simulink model "KillerWhaleModelPneumaticControl"  (R2020b)
settings: Solver=ode15s  StartTime=0.0  StopTime=10  MaxStep=0.01  RelTol=1e-3
model workspace: external: MATLAB File KillerWhaleParams.m (data not in the file)
undefined symbols (not defined in the file or in its folder): frontParams, rearParams, standParams, X, Y, Z
libraries: sm_lib x4301, nesl_utility x6
(part 2 of 66)

== system KillerWhaleModelPneumaticControl/WhaleStand ==
  J5 : Inport
  Cylindrical1 : sm_lib/Joints/Cylindrical Joint  JointMode=Normal  SenseConstraintForce=off  SenseConstraintForceX=off  SenseConstraintForceY=off  SenseConstraintForceZ=off  SenseConstraintTorque=off  SenseConstraintTorqueX=off  SenseConstraintTorqueY=off  SenseConstraintTorqueZ=off  SenseTotalForce=off  SenseTotalForceX=off  SenseTotalForceY=off  SenseTotalForceZ=off  SenseTotalTorque=off  SenseTotalTorqueX=off  SenseTotalTorqueY=off  SenseTotalTorqueZ=off  CompositeWrenchDir=FollowerOnBase  CompositeWrenchFrame=BaseFrame  PzEquilibriumPosition=0  PzEquilibriumPositionUnits=m  PzSpringStiffness=0  PzSpringStiffnessUnits=N/m  PzDampingCoefficient=0  PzDampingCoefficientUnits=N/(m/s)  PzTorqueActuationMode=NoTorque  PzMotionActuationMode=ComputedMotion  PzSensePosition=off  PzSenseVelocity=off  PzSenseAcceleration=off  PzSenseTorqueForce=off  PzSenseLowerLimitTorqueForce=off  PzSenseUpperLimitTorqueForce=off  PzLowerLimitSpecify=off  PzLowerLimitBound=-1  PzLowerLimitBoundUnits=m  PzLowerLimitStiffness=1e6  PzLowerLimitStiffnessUnits=N/m  PzLowerLimitDamping=1e3  PzLowerLimitDampingUnits=N/(m/s)  PzLowerLimitTransitionRegionWidth=1e-4  PzLowerLimitTransitionRegionWidthUnits=m  PzUpperLimitSpecify=off  PzUpperLimitBound=1  PzUpperLimitBoundUnits=m  PzUpperLimitStiffness=1e6  PzUpperLimitStiffnessUnits=N/m  PzUpperLimitDamping=1e3  PzUpperLimitDampingUnits=N/(m/s)  PzUpperLimitTransitionRegionWidth=1e-4  PzUpperLimitTransitionRegionWidthUnits=m  PzPositionTargetSpecify=off  PzPositionTargetPriority=High  PzPositionTargetValue=0  PzPositionTargetValueUnits=m  PzVelocityTargetSpecify=off  PzVelocityTargetPriority=High  PzVelocityTargetValue=0  PzVelocityTargetValueUnits=m/s  RzEquilibriumPosition=0  RzEquilibriumPositionUnits=deg  RzSpringStiffness=0  RzSpringStiffnessUnits=N*m/deg  RzDampingCoefficient=0  RzDampingCoefficientUnits=N*m/(deg/s)  RzTorqueActuationMode=NoTorque  RzMotionActuationMode=ComputedMotion  RzSensePosition=off  RzSenseVelocity=off  RzSenseAcceleration=off  RzSenseTorqueForce=off  RzSenseLowerLimitTorqueForce=off  RzSenseUpperLimitTorqueForce=off  RzLowerLimitSpecify=off  RzLowerLimitBound=-90  RzLowerLimitBoundUnits=deg  RzLowerLimitStiffness=1e4  RzLowerLimitStiffnessUnits=N*m/deg  RzLowerLimitDamping=10  RzLowerLimitDampingUnits=N*m/(deg/s)  RzLowerLimitTransitionRegionWidth=0.1  RzLowerLimitTransitionRegionWidthUnits=deg  RzUpperLimitSpecify=off  RzUpperLimitBound=90  RzUpperLimitBoundUnits=deg  RzUpperLimitStiffness=1e4  RzUpperLimitStiffnessUnits=N*m/deg  RzUpperLimitDamping=10  RzUpperLimitDampingUnits=N*m/(deg/s)  RzUpperLimitTransitionRegionWidth=0.1  RzUpperLimitTransitionRegionWidthUnits=deg  RzPositionTargetSpecify=off  RzPositionTargetPriority=High  RzPositionTargetValue=0  RzPositionTargetValueUnits=deg  RzVelocityTargetSpecify=off  RzVelocityTargetPriority=High  RzVelocityTargetValue=0  RzVelocityTargetValueUnits=deg/s
  Cylindrical2 : sm_lib/Joints/Cylindrical Joint  JointMode=Normal  SenseConstraintForce=off  SenseConstraintForceX=off  SenseConstraintForceY=off  SenseConstraintForceZ=off  SenseConstraintTorque=off  SenseConstraintTorqueX=off  SenseConstraintTorqueY=off  SenseConstraintTorqueZ=off  SenseTotalForce=off  SenseTotalForceX=off  SenseTotalForceY=off  SenseTotalForceZ=off  SenseTotalTorque=off  SenseTotalTorqueX=off  SenseTotalTorqueY=off  SenseTotalTorqueZ=off  CompositeWrenchDir=FollowerOnBase  CompositeWrenchFrame=BaseFrame  PzEquilibriumPosition=0  PzEquilibriumPositionUnits=m  PzSpringStiffness=0  PzSpringStiffnessUnits=N/m  PzDampingCoefficient=0  PzDampingCoefficientUnits=N/(m/s)  PzTorqueActuationMode=NoTorque  PzMotionActuationMode=ComputedMotion  PzSensePosition=off  PzSenseVelocity=off  PzSenseAcceleration=off  PzSenseTorqueForce=off  PzSenseLowerLimitTorqueForce=off  PzSenseUpperLimitTorqueForce=off  PzLowerLimitSpecify=off  PzLowerLimitBound=-1  PzLowerLimitBoundUnits=m  PzLowerLimitStiffness=1e6  PzLowerLimitStiffnessUnits=N/m  PzLowerLimitDamping=1e3  PzLowerLimitDampingUnits=N/(m/s)  PzLowerLimitTransitionRegionWidth=1e-4  PzLowerLimitTransitionRegionWidthUnits=m  PzUpperLimitSpecify=off  PzUpperLimitBound=1  PzUpperLimitBoundUnits=m  PzUpperLimitStiffness=1e6  PzUpperLimitStiffnessUnits=N/m  PzUpperLimitDamping=1e3  PzUpperLimitDampingUnits=N/(m/s)  PzUpperLimitTransitionRegionWidth=1e-4  PzUpperLimitTransitionRegionWidthUnits=m  PzPositionTargetSpecify=off  PzPositionTargetPriority=High  PzPositionTargetValue=0  PzPositionTargetValueUnits=m  PzVelocityTargetSpecify=off  PzVelocityTargetPriority=High  PzVelocityTargetValue=0  PzVelocityTargetValueUnits=m/s  RzEquilibriumPosition=0  RzEquilibriumPositionUnits=deg  RzSpringStiffness=0  RzSpringStiffnessUnits=N*m/deg  RzDampingCoefficient=0  RzDampingCoefficientUnits=N*m/(deg/s)  RzTorqueActuationMode=NoTorque  RzMotionActuationMode=ComputedMotion  RzSensePosition=off  RzSenseVelocity=off  RzSenseAcceleration=off  RzSenseTorqueForce=off  RzSenseLowerLimitTorqueForce=off  RzSenseUpperLimitTorqueForce=off  RzLowerLimitSpecify=off  RzLowerLimitBound=-90  RzLowerLimitBoundUnits=deg  RzLowerLimitStiffness=1e4  RzLowerLimitStiffnessUnits=N*m/deg  RzLowerLimitDamping=10  RzLowerLimitDampingUnits=N*m/(deg/s)  RzLowerLimitTransitionRegionWidth=0.1  RzLowerLimitTransitionRegionWidthUnits=deg  RzUpperLimitSpecify=off  RzUpperLimitBound=90  RzUpperLimitBoundUnits=deg  RzUpperLimitStiffness=1e4  RzUpperLimitStiffnessUnits=N*m/deg  RzUpperLimitDamping=10  RzUpperLimitDampingUnits=N*m/(deg/s)  RzUpperLimitTransitionRegionWidth=0.1  RzUpperLimitTransitionRegionWidthUnits=deg  RzPositionTargetSpecify=off  RzPositionTargetPriority=High  RzPositionTargetValue=0  RzPositionTargetValueUnits=deg  RzVelocityTargetSpecify=off  RzVelocityTargetPriority=High  RzVelocityTargetValue=0  RzVelocityTargetValueUnits=deg/s
  Link_1_1 : Subsystem
  PitchLink2_1 : Subsystem
  PitchLink3_1 : Subsystem
      settings: PortSchema="{\"entries\":[{\"content\":{\"sides\":[{\"content\":{\"connectorIds\":[\"LConn1\"]},\"type\":\"ConnectorPlacement.EquallySpacedRectSide\",\"uuid\":\"a9d62d2a-b569-4d18-acf6-632282cdfd3f\"},{\"content\":{\"connectorIds\":[\"RConn1\"],\"side\":\"RIGHT\"},\"type\":\"ConnectorPlacement.EquallySpacedRectSide\",\"uuid\":\"ddf08f5b-84f7-435f-8135-0f34e66a3f6c\"},{\"content\":{\"connectorIds\":[\"LConn2\"],\"side\":\"TOP\"},\"type\":\"ConnectorPlacement.EquallySpacedRectSide\",\"uuid\":\"528ea33a-f0b8-4f6d-8194-a808427dd81b\"},{\"content\":{\"connectorIds\":[],\"side\":\"HIDDEN\"},\"type\":\"ConnectorPlacement.EquallySpacedRectSide\",\"uuid\":\"99e749ff-748c-40e2-8d76-9e8f4512f99c\"}]},\"type\":\"ConnectorPlacement.EquallySpacedConnector\",\"uuid\":\"82bcbf93-e613-46bd-8073-2373def69e08\"}],\"packageUris\":[\"http://schema.mathworks.com/mf0/Connector/R2020b\"],\"version\":\"1.0\"}"
  PitchLink4_1 : Subsystem
  Revolute1 : sm_lib/Joints/Revolute Joint  JointMode=Normal  SenseConstraintForce=off  SenseConstraintForceX=off  SenseConstraintForceY=off  SenseConstraintForceZ=off  SenseConstraintTorque=off  SenseConstraintTorqueX=off  SenseConstraintTorqueY=off  SenseConstraintTorqueZ=off  SenseTotalForce=off  SenseTotalForceX=off  SenseTotalForceY=off  SenseTotalForceZ=off  SenseTotalTorque=off  SenseTotalTorqueX=off  SenseTotalTorqueY=off  SenseTotalTorqueZ=off  CompositeWrenchDir=FollowerOnBase  CompositeWrenchFrame=BaseFrame  EquilibriumPosition=0  EquilibriumPositionUnits=deg  SpringStiffness=0  SpringStiffnessUnits=N*m/deg  DampingCoefficient=0  DampingCoefficientUnits=N*m/(deg/s)  TorqueActuationMode=NoTorque  MotionActuationMode=ComputedMotion  SensePosition=off  SenseVelocity=off  SenseAcceleration=off  SenseTorqueForce=off  SenseLowerLimitTorqueForce=off  SenseUpperLimitTorqueForce=off  LowerLimitSpecify=off  LowerLimitBound=-90  LowerLimitBoundUnits=deg  LowerLimitStiffness=1e4  LowerLimitStiffnessUnits=N*m/deg  LowerLimitDamping=10  LowerLimitDampingUnits=N*m/(deg/s)  LowerLimitTransitionRegionWidth=0.1  LowerLimitTransitionRegionWidthUnits=deg  UpperLimitSpecify=off  UpperLimitBound=90  UpperLimitBoundUnits=deg  UpperLimitStiffness=1e4  UpperLimitStiffnessUnits=N*m/deg  UpperLimitDamping=10  UpperLimitDampingUnits=N*m/(deg/s)  UpperLimitTransitionRegionWidth=0.1  UpperLimitTransitionRegionWidthUnits=deg  PositionTargetSpecify=on  PositionTargetPriority=Low  PositionTargetValue=standParams.RevoluteJoint(2).Rz.Pos  PositionTargetValueUnits=deg  VelocityTargetSpecify=off  VelocityTargetPriority=High  VelocityTargetValue=0  VelocityTargetValueUnits=deg/s
  Revolute2 : sm_lib/Joints/Revolute Joint  JointMode=Normal  SenseConstraintForce=off  SenseConstraintForceX=off  SenseConstraintForceY=off  SenseConstraintForceZ=off  SenseConstraintTorque=off  SenseConstraintTorqueX=off  SenseConstraintTorqueY=off  SenseConstraintTorqueZ=off  SenseTotalForce=off  SenseTotalForceX=off  SenseTotalForceY=off  SenseTotalForceZ=off  SenseTotalTorque=off  SenseTotalTorqueX=off  SenseTotalTorqueY=off  SenseTotalTorqueZ=off  CompositeWrenchDir=FollowerOnBase  CompositeWrenchFrame=BaseFrame  EquilibriumPosition=0  EquilibriumPositionUnits=deg  SpringStiffness=0  SpringStiffnessUnits=N*m/deg  DampingCoefficient=0  DampingCoefficientUnits=N*m/(deg/s)  TorqueActuationMode=NoTorque  MotionActuationMode=ComputedMotion  SensePosition=off  SenseVelocity=off  SenseAcceleration=off  SenseTorqueForce=off  SenseLowerLimitTorqueForce=off  SenseUpperLimitTorqueForce=off  LowerLimitSpecify=off  LowerLimitBound=-90  LowerLimitBoundUnits=deg  LowerLimitStiffness=1e4  LowerLimitStiffnessUnits=N*m/deg  LowerLimitDamping=10  LowerLimitDampingUnits=N*m/(deg/s)  LowerLimitTransitionRegionWidth=0.1  LowerLimitTransitionRegionWidthUnits=deg  UpperLimitSpecify=off  UpperLimitBound=90  UpperLimitBoundUnits=deg  UpperLimitStiffness=1e4  UpperLimitStiffnessUnits=N*m/deg  UpperLimitDamping=10  UpperLimitDampingUnits=N*m/(deg/s)  UpperLimitTransitionRegionWidth=0.1  UpperLimitTransitionRegionWidthUnits=deg  PositionTargetSpecify=on  PositionTargetPriority=Low  PositionTargetValue=standParams.RevoluteJoint(3).Rz.Pos  PositionTargetValueUnits=deg  VelocityTargetSpecify=off  VelocityTargetPriority=High  VelocityTargetValue=0  VelocityTargetValueUnits=deg/s
  Revolute3 : sm_lib/Joints/Revolute Joint  JointMode=Normal  SenseConstraintForce=off  SenseConstraintForceX=off  SenseConstraintForceY=off  SenseConstraintForceZ=off  SenseConstraintTorque=off  SenseConstraintTorqueX=off  SenseConstraintTorqueY=off  SenseConstraintTorqueZ=off  SenseTotalForce=off  SenseTotalForceX=off  SenseTotalForceY=off  SenseTotalForceZ=off  SenseTotalTorque=off  SenseTotalTorqueX=off  SenseTotalTorqueY=off  SenseTotalTorqueZ=off  CompositeWrenchDir=FollowerOnBase  CompositeWrenchFrame=BaseFrame  EquilibriumPosition=0  EquilibriumPositionUnits=deg  SpringStiffness=0  SpringStiffnessUnits=N*m/deg  DampingCoefficient=0  DampingCoefficientUnits=N*m/(deg/s)  TorqueActuationMode=NoTorque  MotionActuationMode=ComputedMotion  SensePosition=off  SenseVelocity=off  SenseAcceleration=off  SenseTorqueForce=off  SenseLowerLimitTorqueForce=off  SenseUpperLimitTorqueForce=off  LowerLimitSpecify=off  LowerLimitBound=-90  LowerLimitBoundUnits=deg  LowerLimitStiffness=1e4  LowerLimitStiffnessUnits=N*m/deg  LowerLimitDamping=10  LowerLimitDampingUnits=N*m/(deg/s)  LowerLimitTransitionRegionWidth=0.1  LowerLimitTransitionRegionWidthUnits=deg  UpperLimitSpecify=off  UpperLimitBound=90  UpperLimitBoundUnits=deg  UpperLimitStiffness=1e4  UpperLimitStiffnessUnits=N*m/deg  UpperLimitDamping=10  UpperLimitDampingUnits=N*m/(deg/s)  UpperLimitTransitionRegionWidth=0.1  UpperLimitTransitionRegionWidthUnits=deg  PositionTargetSpecify=on  PositionTargetPriority=Low  PositionTargetValue=standParams.RevoluteJoint(5).Rz.Pos  PositionTargetValueUnits=deg  VelocityTargetSpecify=off  VelocityTargetPriority=High  VelocityTargetValue=0  VelocityTargetValueUnits=deg/s
  Revolute4 : sm_lib/Joints/Revolute Joint  JointMode=Normal  SenseConstraintForce=off  SenseConstraintForceX=off  SenseConstraintForceY=off  SenseConstraintForceZ=off  SenseConstraintTorque=off  SenseConstraintTorqueX=off  SenseConstraintTorqueY=off  SenseConstraintTorqueZ=off  SenseTotalForce=off  SenseTotalForceX=off  SenseTotalForceY=off  SenseTotalForceZ=off  SenseTotalTorque=off  SenseTotalTorqueX=off  SenseTotalTorqueY=off  SenseTotalTorqueZ=off  CompositeWrenchDir=FollowerOnBase  CompositeWrenchFrame=BaseFrame  EquilibriumPosition=0  EquilibriumPositionUnits=deg  SpringStiffness=0  SpringStiffnessUnits=N*m/deg  DampingCoefficient=0  DampingCoefficientUnits=N*m/(deg/s)  TorqueActuationMode=NoTorque  MotionActuationMode=ComputedMotion  SensePosition=off  SenseVelocity=off  SenseAcceleration=off  SenseTorqueForce=off  SenseLowerLimitTorqueForce=off  SenseUpperLimitTorqueForce=off  LowerLimitSpecify=off  LowerLimitBound=-90  LowerLimitBoundUnits=deg  LowerLimitStiffness=1e4  LowerLimitStiffnessUnits=N*m/deg  LowerLimitDamping=10  LowerLimitDampingUnits=N*m/(deg/s)  LowerLimitTransitionRegionWidth=0.1  LowerLimitTransitionRegionWidthUnits=deg  UpperLimitSpecify=off  UpperLimitBound=90  UpperLimitBoundUnits=deg  UpperLimitStiffness=1e4  UpperLimitStiffnessUnits=N*m/deg  UpperLimitDamping=10  UpperLimitDampingUnits=N*m/(deg/s)  UpperLimitTransitionRegionWidth=0.1  UpperLimitTransitionRegionWidthUnits=deg  PositionTargetSpecify=on  PositionTargetPriority=Low  PositionTargetValue=standParams.RevoluteJoint(1).Rz.Pos  PositionTargetValueUnits=deg  VelocityTargetSpecify=off  VelocityTargetPriority=High  VelocityTargetValue=0  VelocityTargetValueUnits=deg/s
  Revolute5 : sm_lib/Joints/Revolute Joint  JointMode=Normal  SenseConstraintForce=off  SenseConstraintForceX=off  SenseConstraintForceY=off  SenseConstraintForceZ=off  SenseConstraintTorque=off  SenseConstraintTorqueX=off  SenseConstraintTorqueY=off  SenseConstraintTorqueZ=off  SenseTotalForce=off  SenseTotalForceX=off  SenseTotalForceY=off  SenseTotalForceZ=off  SenseTotalTorque=off  SenseTotalTorqueX=off  SenseTotalTorqueY=off  SenseTotalTorqueZ=off  CompositeWrenchDir=FollowerOnBase  CompositeWrenchFrame=BaseFrame  EquilibriumPosition=0  EquilibriumPositionUnits=deg  SpringStiffness=0  SpringStiffnessUnits=N*m/deg  DampingCoefficient=0  DampingCoefficientUnits=N*m/(deg/s)  TorqueActuationMode=NoTorque  MotionActuationMode=ComputedMotion  SensePosition=off  SenseVelocity=off  SenseAcceleration=off  SenseTorqueForce=off  SenseLowerLimitTorqueForce=off  SenseUpperLimitTorqueForce=off  LowerLimitSpecify=off  LowerLimitBound=-90  LowerLimitBoundUnits=deg  LowerLimitStiffness=1e4  LowerLimitStiffnessUnits=N*m/deg  LowerLimitDamping=10  LowerLimitDampingUnits=N*m/(deg/s)  LowerLimitTransitionRegionWidth=0.1  LowerLimitTransitionRegionWidthUnits=deg  UpperLimitSpecify=off  UpperLimitBound=90  UpperLimitBoundUnits=deg  UpperLimitStiffness=1e4  UpperLimitStiffnessUnits=N*m/deg  UpperLimitDamping=10  UpperLimitDampingUnits=N*m/(deg/s)  UpperLimitTransitionRegionWidth=0.1  UpperLimitTransitionRegionWidthUnits=deg  PositionTargetSpecify=on  PositionTargetPriority=Low  PositionTargetValue=standParams.RevoluteJoint(4).Rz.Pos  PositionTargetValueUnits=deg  VelocityTargetSpecify=off  VelocityTargetPriority=High  VelocityTargetValue=0  VelocityTargetValueUnits=deg/s
  Stand_1 : Subsystem
  Stand_Actuator_1 : Subsystem
      settings: PortSchema="{\"entries\":[{\"content\":{\"sides\":[{\"content\":{\"connectorIds\":[\"LConn1\"]},\"type\":\"ConnectorPlacement.EquallySpacedRectSide\",\"uuid\":\"a2790423-1875-4f6c-bcc8-f8951bbf04a9\"},{\"content\":{\"connectorIds\":[\"RConn1\"],\"side\":\"RIGHT\"},\"type\":\"ConnectorPlacement.EquallySpacedRectSide\",\"uuid\":\"c84b9fae-4c29-439d-9486-1840c3d66b05\"},{\"content\":{\"connectorIds\":[\"In1\"],\"side\":\"TOP\"},\"type\":\"ConnectorPlacement.EquallySpacedRectSide\",\"uuid\":\"97f54a40-5d41-49e0-a709-056e005671f1\"},{\"content\":{\"connectorIds\":[],\"side\":\"HIDDEN\"},\"type\":\"ConnectorPlacement.EquallySpacedRectSide\",\"uuid\":\"427997b4-744f-45dd-b609-16314c135bf0\"}]},\"type\":\"ConnectorPlacement.EquallySpacedConnector\",\"uuid\":\"a7b9e3e0-830a-4064-b5fb-feaf5802e4ca\"}],\"packageUris\":[\"http://schema.mathworks.com/mf0/Connector/R2020b\"],\"version\":\"1.0\"}"
  Transform : sm_lib/Frames and Transforms/Rigid Transform  TranslationMethod=Cartesian  TranslationStandardOffset=0  TranslationLengthUnit=in  TranslationStandardAxis=+Z  TranslationCartesianOffset=standParams.RigidTransform(321).translation  TranslationROffset=0  TranslationROffsetUnits=m  TranslationZOffset=0  TranslationZOffsetUnits=m  TranslationThetaOffset=0  TranslationThetaOffsetUnits=deg  RotationMethod=ArbitraryAxis  RotationAngleUnits=rad  RotationStandardAxis=+Z  RotationAngle=standParams.RigidTransform(321).angle  RotationArbitraryAxis=standParams.RigidTransform(321).axis  FollAlignAxisA=+X  BaseAlignAxisA=+Y  FollAlignAxisB=+Y  BaseAlignAxisB=+Z  RotationSequenceAxes=FollowerAxes  RotationSequence=XYX  RotationSequenceAngles=[0 0 0]  RotationSequenceAnglesUnits=deg  RotationMatrix=[1 0 0; 0 1 0; 0 0 1]
  S1 : PMIOPort  Side=Left
  S2 : PMIOPort  Port=2  Side=Left
  wires:
  J5/1 -> Stand_Actuator_1/1(J5)
  connections:
  Cylindrical2/LConn1 -- Stand_Actuator_1/RConn1
  Revolute5/RConn1 -- Stand_Actuator_1/LConn1
  Cylindrical1/RConn1 -- Link_1_1/LConn2
  PitchLink3_1/LConn1 -- Revolute3/RConn1
  PitchLink3_1/RConn1 -- Revolute1/LConn1
  Revolute5/LConn1 -- Stand_1/RConn1
  PitchLink4_1/LConn1 -- Revolute4/RConn1
  PitchLink2_1/RConn2 -- Revolute2/LConn1
  Cylindrical2/RConn1 -- Link_1_1/LConn1
  Cylindrical1/LConn1 -- Stand_1/RConn2
  Transform/RConn1 -- Stand_1/LConn1
  Revolute4/LConn1 -- Stand_1/RConn3
  PitchLink4_1/LConn2 -- Revolute1/RConn1
  Link_1_1/LConn3 -- Revolute2/RConn1
  PitchLink2_1/RConn1 -- Revolute3/LConn1
  S2/RConn1 -- Transform/LConn1
  S1/RConn1 -- PitchLink3_1/LConn2

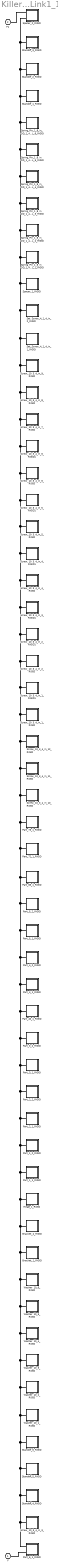
== system KillerWhaleModelPneumaticControl/HeadLinkage/HeadLink1_1 ==
  Bracket_1_RIGID : Subsystem
  Bracket_2_RIGID : Subsystem
  Hinge_1_RIGID : Subsystem
  Part_1_1_RIGID : Subsystem
  Part_1_2_RIGID : Subsystem
  Part_2_1_RIGID : Subsystem
  Part_2_2_RIGID : Subsystem
  Part_3_1_RIGID : Subsystem
  Part_3_2_RIGID : Subsystem
  Part_40_1_RIGID : Subsystem
  Part_4_1_RIGID : Subsystem
  Part_4_2_RIGID : Subsystem
  Part_5_1_RIGID : Subsystem
  Part_5_2_RIGID : Subsystem
  Part_65_1_RIGID : Subsystem
  Part_6_1_RIGID : Subsystem
  Part_72_1_RIGID : Subsystem
  Part_73_1_RIGID : Subsystem
  Screw_10_3_4_in_10_RIGID : Subsystem
  Screw_10_3_4_in_11_RIGID : Subsystem
  Screw_10_3_4_in_12_RIGID : Subsystem
  Screw_10_3_4_in_1_RIGID : Subsystem
  Screw_10_3_4_in_1_RIGID1 : Subsystem
  Screw_10_3_4_in_2_RIGID : Subsystem
  Screw_10_3_4_in_2_RIGID1 : Subsystem
  Screw_10_3_4_in_3_RIGID : Subsystem
  Screw_10_3_4_in_3_RIGID1 : Subsystem
  Screw_10_3_4_in_4_RIGID : Subsystem
  Screw_10_3_4_in_4_RIGID1 : Subsystem
  Screw_10_3_4_in_5_RIGID : Subsystem
  Screw_10_3_4_in_5_RIGID1 : Subsystem
  Screw_10_3_4_in_6_RIGID : Subsystem
  Screw_10_3_4_in_6_RIGID1 : Subsystem
  Screw_10_3_4_in_7_RIGID : Subsystem
  Screw_10_3_4_in_8_RIGID : Subsystem
  Screw_10_3_4_in_9_RIGID : Subsystem
  Set_Screw_4_1_4_in_1_RIGID : Subsystem
  Set_Screw_4_1_4_in_2_RIGID : Subsystem
  Spacer_1_RIGID : Subsystem
  Spacer_2_RIGID : Subsystem
  Spring_Pin_1_8_in_OD_1_4_in_L_1_RIGID : Subsystem
  Spring_Pin_1_8_in_OD_1_4_in_L_2_RIGID : Subsystem
  Spring_Pin_1_8_in_OD_1_4_in_L_3_RIGID : Subsystem
  Spring_Pin_1_8_in_OD_1_4_in_L_4_RIGID : Subsystem
  Spring_Pin_1_8_in_OD_1_4_in_L_5_RIGID : Subsystem
  Spring_Pin_1_8_in_OD_1_4_in_L_6_RIGID : Subsystem
  Standoff_1_RIGID : Subsystem
  Standoff_2_RIGID : Subsystem
  Standoff_3_RIGID : Subsystem
  Standoff_4_RIGID : Subsystem
  Standoff_5_RIGID : Subsystem
  Standoff_6_RIGID : Subsystem
  Washer_10_1_RIGID : Subsystem
  Washer_10_2_RIGID : Subsystem
  Washer_10_3_RIGID : Subsystem
  Washer_10_4_RIGID : Subsystem
  Washer_10_5_RIGID : Subsystem
  Washer_10_6_RIGID : Subsystem
  F : PMIOPort  Side=Left
  F1 : PMIOPort  Port=2  Side=Right
  connections:
  Bracket_1_RIGID/LConn1 -- Part_6_1_RIGID/LConn1 -- Screw_10_3_4_in_3_RIGID/LConn1 -- Standoff_4_RIGID/LConn1 -- Standoff_5_RIGID/LConn1 -- Standoff_6_RIGID/LConn1 -- Washer_10_1_RIGID/LConn1 -- Washer_10_2_RIGID/LConn1 -- Washer_10_3_RIGID/LConn1 -- Washer_10_4_RIGID/LConn1 -- Washer_10_5_RIGID/LConn1 -- Washer_10_6_RIGID/LConn1 -- Spacer_2_RIGID/LConn2 -- Standoff_3_RIGID/LConn1 -- Standoff_2_RIGID/LConn1 -- Standoff_1_RIGID/LConn1 -- Spring_Pin_1_8_in_OD_1_4_in_L_6_RIGID/LConn1 -- Spring_Pin_1_8_in_OD_1_4_in_L_5_RIGID/LConn1 -- Spring_Pin_1_8_in_OD_1_4_in_L_4_RIGID/LConn1 -- Spring_Pin_1_8_in_OD_1_4_in_L_3_RIGID/LConn1 -- Spring_Pin_1_8_in_OD_1_4_in_L_2_RIGID/LConn1 -- Spring_Pin_1_8_in_OD_1_4_in_L_1_RIGID/LConn1 -- Spacer_1_RIGID/LConn1 -- Set_Screw_4_1_4_in_2_RIGID/LConn1 -- Set_Screw_4_1_4_in_1_RIGID/LConn1 -- Screw_10_3_4_in_9_RIGID/LConn1 -- Screw_10_3_4_in_8_RIGID/LConn1 -- Screw_10_3_4_in_7_RIGID/LConn1 -- Screw_10_3_4_in_6_RIGID1/LConn1 -- Screw_10_3_4_in_6_RIGID/LConn1 -- Screw_10_3_4_in_5_RIGID1/LConn1 -- Screw_10_3_4_in_5_RIGID/LConn1 -- Screw_10_3_4_in_4_RIGID1/LConn1 -- Screw_10_3_4_in_4_RIGID/LConn1 -- Screw_10_3_4_in_3_RIGID1/LConn1 -- Screw_10_3_4_in_2_RIGID1/LConn1 -- Screw_10_3_4_in_2_RIGID/LConn1 -- Screw_10_3_4_in_1_RIGID1/LConn1 -- Screw_10_3_4_in_1_RIGID/LConn1 -- Screw_10_3_4_in_12_RIGID/LConn1 -- Screw_10_3_4_in_11_RIGID/LConn1 -- Screw_10_3_4_in_10_RIGID/LConn1 -- Part_73_1_RIGID/LConn1 -- Part_72_1_RIGID/LConn1 -- Part_65_1_RIGID/LConn1 -- Part_5_2_RIGID/LConn1 -- Part_5_1_RIGID/LConn1 -- Part_4_2_RIGID/LConn1 -- Part_4_1_RIGID/LConn1 -- Part_40_1_RIGID/LConn1 -- Part_3_2_RIGID/LConn1 -- Part_3_1_RIGID/LConn1 -- Part_2_2_RIGID/LConn1 -- Part_2_1_RIGID/LConn1 -- Part_1_2_RIGID/LConn1 -- Part_1_1_RIGID/LConn1 -- Hinge_1_RIGID/LConn1 -- Bracket_2_RIGID/LConn1
  Part_6_1_RIGID/LConn2 -- F/RConn1
  Spacer_2_RIGID/LConn1 -- F1/RConn1

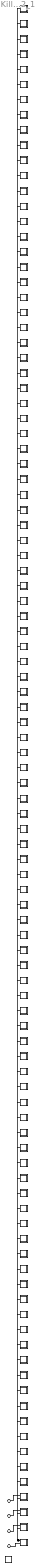
== system KillerWhaleModelPneumaticControl/HeadLinkage/HeadLink2_1 ==
  Frame_Part_1_RIGID : Subsystem
  Frame_Part_2_RIGID : Subsystem
  Part_1_1_RIGID : Subsystem
  Part_1_2_RIGID : Subsystem
  Part_1_3_RIGID : Subsystem
  Part_1_4_RIGID : Subsystem
  Part_24_1_RIGID : Subsystem
  Part_24r_1_RIGID : Subsystem
  Part_2_1_RIGID : Subsystem
  Part_2_2_RIGID : Subsystem
  Part_2_3_RIGID : Subsystem
  Part_2_4_RIGID : Subsystem
  Part_3_1_RIGID : Subsystem
  Part_3_2_RIGID : Subsystem
  Part_3_3_RIGID : Subsystem
  Part_3_4_RIGID : Subsystem
  Part_4_1_RIGID : Subsystem
  Part_4_2_RIGID : Subsystem
  Part_4_3_RIGID : Subsystem
  Part_4_4_RIGID : Subsystem
  Part_5_1_RIGID : Subsystem
  Part_5_2_RIGID : Subsystem
  Part_5_3_RIGID : Subsystem
  Part_5_4_RIGID : Subsystem
  Part_6_1_RIGID : Subsystem
  Part_6_2_RIGID : Subsystem
  Part_809_1_RIGID : Subsystem
  Part_809_2_RIGID : Subsystem
  Part_809_3_RIGID : Subsystem
  Part_809_4_RIGID : Subsystem
  Part_809_5_RIGID : Subsystem
  Part_811_1_RIGID : Subsystem
  Part_812_1_RIGID : Subsystem
  Part_813_1_RIGID : Subsystem
  Part_814_1_RIGID : Subsystem
  Part_815_1_RIGID : Subsystem
  Part_816_1_RIGID : Subsystem
  Part_817_1_RIGID : Subsystem
  Part_818_1_RIGID : Subsystem
  Part_819_1_RIGID : Subsystem
  Part_820_1_RIGID : Subsystem
  Part_821_1_RIGID : Subsystem
  Part_822_1_RIGID : Subsystem
  Part_823_1_RIGID : Subsystem
  Part_824_1_RIGID : Subsystem
  Part_824_2_RIGID : Subsystem
  Part_825_1_RIGID : Subsystem
  Part_825_2_RIGID : Subsystem
  Part_826_1_RIGID : Subsystem
  Part_826_2_RIGID : Subsystem
  Part_827_1_RIGID : Subsystem
  Part_827_2_RIGID : Subsystem
  Part_828_1_RIGID : Subsystem
  Part_828_2_RIGID : Subsystem
  Part_867_1_RIGID : Subsystem
  Part_870_1_RIGID : Subsystem
  Part_875_1_RIGID : Subsystem
  Part_936_1_RIGID : Subsystem
  Part_937_1_RIGID : Subsystem
  Part_938_1_RIGID : Subsystem
  Part_939_1_RIGID : Subsystem
  ReferenceFrame : sm_lib/Frames and Transforms/Reference Frame
  Screw_10_3_4_in_1_RIGID : Subsystem
  Screw_10_3_4_in_2_RIGID : Subsystem
  Screw_10_3_4_in_3_RIGID : Subsystem
  Screw_10_3_4_in_4_RIGID : Subsystem
  Screw_10_3_4_in_5_RIGID : Subsystem
  Screw_10_3_4_in_6_RIGID : Subsystem
  Screw_8_1_2_in_1_RIGID : Subsystem
  Screw_8_1_2_in_2_RIGID : Subsystem
  Spring_Pin_1_8_in_OD_1_4_in_L_1_RIGID : Subsystem
  Spring_Pin_1_8_in_OD_1_4_in_L_2_RIGID : Subsystem
  Spring_Pin_1_8_in_OD_1_4_in_L_3_RIGID : Subsystem
  Spring_Pin_1_8_in_OD_1_4_in_L_4_RIGID : Subsystem
  Spring_Pin_1_8_in_OD_1_4_in_L_5_RIGID : Subsystem
  Spring_Pin_1_8_in_OD_1_4_in_L_6_RIGID : Subsystem
  Standoff_1_RIGID : Subsystem
  Washer_10_10_RIGID : Subsystem
  Washer_10_1_RIGID : Subsystem
  Washer_10_2_RIGID : Subsystem
  Washer_10_3_RIGID : Subsystem
  Washer_10_4_RIGID : Subsystem
  Washer_10_5_RIGID : Subsystem
  Washer_10_6_RIGID : Subsystem
  Washer_10_7_RIGID : Subsystem
  Washer_10_8_RIGID : Subsystem
  Washer_10_9_RIGID : Subsystem
  Washer_8_1_RIGID : Subsystem
  Washer_8_2_RIGID : Subsystem
  bulkheads7_1_RIGID : Subsystem
  bulkheads7_2_RIGID : Subsystem
  bulkheads7_3_RIGID : Subsystem
  bulkheads7_4_RIGID : Subsystem
  bulkheads7_5_RIGID : Subsystem
  bulkheads8_1_RIGID : Subsystem
  bulkheads8_2_RIGID : Subsystem
  bulkheads8_3_RIGID : Subsystem
  bulkheads8_4_RIGID : Subsystem
  bulkheads8_5_RIGID : Subsystem
  nut_1_RIGID : Subsystem
  nut_2_RIGID : Subsystem
  nut_3_RIGID : Subsystem
  nut_4_RIGID : Subsystem
  F2 : PMIOPort  Side=Left
  F1 : PMIOPort  Port=2  Side=Left
  F4 : PMIOPort  Port=3  Side=Right
  F : PMIOPort  Port=4  Side=Right
  connections:
  Frame_Part_1_RIGID/LConn1 -- Frame_Part_2_RIGID/LConn2 -- Part_1_1_RIGID/LConn1 -- Part_1_2_RIGID/LConn1 -- Part_1_3_RIGID/LConn2 -- Part_1_4_RIGID/LConn2 -- Part_24_1_RIGID/LConn1 -- Part_24r_1_RIGID/LConn1 -- Part_2_1_RIGID/LConn1 -- Part_2_2_RIGID/LConn1 -- Part_2_3_RIGID/LConn1 -- Part_2_4_RIGID/LConn1 -- Part_3_1_RIGID/LConn1 -- Part_3_2_RIGID/LConn1 -- Part_3_3_RIGID/LConn1 -- Part_3_4_RIGID/LConn1 -- Part_4_1_RIGID/LConn1 -- Part_4_2_RIGID/LConn1 -- Part_4_3_RIGID/LConn1 -- Part_4_4_RIGID/LConn1 -- Part_5_1_RIGID/LConn1 -- Part_5_2_RIGID/LConn1 -- Part_5_3_RIGID/LConn1 -- Part_5_4_RIGID/LConn1 -- Part_6_1_RIGID/LConn1 -- Part_6_2_RIGID/LConn1 -- Part_809_1_RIGID/LConn1 -- Part_809_2_RIGID/LConn1 -- Part_809_3_RIGID/LConn1 -- Part_809_4_RIGID/LConn1 -- Part_809_5_RIGID/LConn1 -- Part_811_1_RIGID/LConn1 -- Part_812_1_RIGID/LConn1 -- Part_813_1_RIGID/LConn1 -- Part_814_1_RIGID/LConn1 -- Part_815_1_RIGID/LConn1 -- Part_816_1_RIGID/LConn1 -- Part_817_1_RIGID/LConn1 -- Part_818_1_RIGID/LConn1 -- Part_819_1_RIGID/LConn1 -- Part_820_1_RIGID/LConn1 -- Part_821_1_RIGID/LConn1 -- Part_822_1_RIGID/LConn1 -- Part_823_1_RIGID/LConn1 -- Part_824_1_RIGID/LConn1 -- Part_824_2_RIGID/LConn1 -- Part_825_1_RIGID/LConn1 -- Part_825_2_RIGID/LConn1 -- Part_826_1_RIGID/LConn1 -- Part_826_2_RIGID/LConn1 -- Part_827_1_RIGID/LConn1 -- Part_827_2_RIGID/LConn1 -- Part_828_1_RIGID/LConn1 -- Part_828_2_RIGID/LConn1 -- Part_867_1_RIGID/LConn1 -- Part_870_1_RIGID/LConn1 -- Part_875_1_RIGID/LConn1 -- Part_936_1_RIGID/LConn1 -- Part_937_1_RIGID/LConn1 -- Part_938_1_RIGID/LConn1 -- Part_939_1_RIGID/LConn1 -- Screw_10_3_4_in_1_RIGID/LConn1 -- Screw_10_3_4_in_2_RIGID/LConn1 -- Screw_10_3_4_in_3_RIGID/LConn1 -- Screw_10_3_4_in_4_RIGID/LConn1 -- Screw_10_3_4_in_5_RIGID/LConn1 -- Screw_10_3_4_in_6_RIGID/LConn1 -- Screw_8_1_2_in_1_RIGID/LConn1 -- Screw_8_1_2_in_2_RIGID/LConn1 -- Spring_Pin_1_8_in_OD_1_4_in_L_1_RIGID/LConn1 -- Spring_Pin_1_8_in_OD_1_4_in_L_2_RIGID/LConn1 -- Spring_Pin_1_8_in_OD_1_4_in_L_3_RIGID/LConn1 -- Spring_Pin_1_8_in_OD_1_4_in_L_4_RIGID/LConn1 -- Spring_Pin_1_8_in_OD_1_4_in_L_5_RIGID/LConn1 -- Spring_Pin_1_8_in_OD_1_4_in_L_6_RIGID/LConn1 -- Standoff_1_RIGID/LConn1 -- Washer_10_10_RIGID/LConn1 -- Washer_10_1_RIGID/LConn1 -- Washer_10_2_RIGID/LConn1 -- Washer_10_3_RIGID/LConn1 -- Washer_10_4_RIGID/LConn1 -- Washer_10_5_RIGID/LConn1 -- Washer_10_6_RIGID/LConn1 -- Washer_10_7_RIGID/LConn1 -- Washer_10_8_RIGID/LConn1 -- Washer_10_9_RIGID/LConn1 -- Washer_8_1_RIGID/LConn1 -- Washer_8_2_RIGID/LConn1 -- bulkheads7_1_RIGID/LConn1 -- bulkheads7_2_RIGID/LConn1 -- bulkheads7_3_RIGID/LConn1 -- bulkheads7_4_RIGID/LConn1 -- bulkheads7_5_RIGID/LConn1 -- bulkheads8_1_RIGID/LConn1 -- bulkheads8_2_RIGID/LConn1 -- bulkheads8_3_RIGID/LConn1 -- bulkheads8_4_RIGID/LConn1 -- bulkheads8_5_RIGID/LConn1 -- nut_1_RIGID/LConn1 -- nut_2_RIGID/LConn1 -- nut_3_RIGID/LConn1 -- nut_4_RIGID/LConn1
  Part_1_4_RIGID/LConn1 -- F/RConn1
  Frame_Part_1_RIGID/LConn2 -- F1/RConn1
  Frame_Part_2_RIGID/LConn1 -- F2/RConn1
  Part_1_3_RIGID/LConn1 -- F4/RConn1

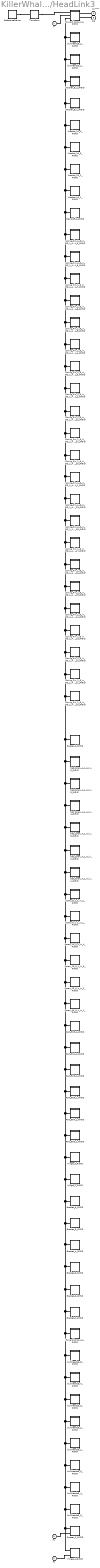
== system KillerWhaleModelPneumaticControl/HeadLinkage/HeadLink3_1 ==
  Bracket_1_RIGID : Subsystem
  Bracket_2_RIGID : Subsystem
  Bracket_3_RIGID : Subsystem
  Bracket_4_RIGID : Subsystem
  Bracket_5_RIGID : Subsystem
  Bracket_6_RIGID : Subsystem
  Hinge_1_RIGID : Subsystem
  Hinge_2_RIGID : Subsystem
  Hinge_3_RIGID : Subsystem
  Part_853_1_RIGID : Subsystem
  Part_854_1_RIGID : Subsystem
  Part_855_1_RIGID : Subsystem
  Part_923_1_RIGID : Subsystem
  Part_924_1_RIGID : Subsystem
  Part_925_1_RIGID : Subsystem
  ReferenceFrame : sm_lib/Frames and Transforms/Reference Frame
  Screw_10_3_4_in_1_RIGID : Subsystem
  Screw_10_3_4_in_2_RIGID : Subsystem
  Screw_10_3_4_in_3_RIGID : Subsystem
  Screw_10_3_4_in_4_RIGID : Subsystem
  Screw_8_1_2_in_1_RIGID : Subsystem
  Screw_8_1_2_in_2_RIGID : Subsystem
  Set_Screw_4_1_4_in_1_RIGID : Subsystem
  Set_Screw_4_1_4_in_2_RIGID : Subsystem
  Set_Screw_4_1_4_in_3_RIGID : Subsystem
  Set_Screw_4_1_4_in_4_RIGID : Subsystem
  Set_Screw_4_1_4_in_5_RIGID : Subsystem
  Set_Screw_4_1_4_in_6_RIGID : Subsystem
  Spacer_1_RIGID : Subsystem
  Spacer_2_RIGID : Subsystem
  Spring_Pin_1_8_in_OD_1_4_in_L_10_RIGID : Subsystem
  Spring_Pin_1_8_in_OD_1_4_in_L_11_RIGID : Subsystem
  Spring_Pin_1_8_in_OD_1_4_in_L_12_RIGID : Subsystem
  Spring_Pin_1_8_in_OD_1_4_in_L_13_RIGID : Subsystem
  Spring_Pin_1_8_in_OD_1_4_in_L_14_RIGID : Subsystem
  Spring_Pin_1_8_in_OD_1_4_in_L_15_RIGID : Subsystem
  Spring_Pin_1_8_in_OD_1_4_in_L_16_RIGID : Subsystem
  Spring_Pin_1_8_in_OD_1_4_in_L_17_RIGID : Subsystem
  Spring_Pin_1_8_in_OD_1_4_in_L_18_RIGID : Subsystem
  Spring_Pin_1_8_in_OD_1_4_in_L_19_RIGID : Subsystem
  Spring_Pin_1_8_in_OD_1_4_in_L_1_RIGID : Subsystem
  Spring_Pin_1_8_in_OD_1_4_in_L_20_RIGID : Subsystem
  Spring_Pin_1_8_in_OD_1_4_in_L_21_RIGID : Subsystem
  Spring_Pin_1_8_in_OD_1_4_in_L_22_RIGID : Subsystem
  Spring_Pin_1_8_in_OD_1_4_in_L_2_RIGID : Subsystem
  Spring_Pin_1_8_in_OD_1_4_in_L_3_RIGID : Subsystem
  Spring_Pin_1_8_in_OD_1_4_in_L_4_RIGID : Subsystem
  Spring_Pin_1_8_in_OD_1_4_in_L_5_RIGID : Subsystem
  Spring_Pin_1_8_in_OD_1_4_in_L_6_RIGID : Subsystem
  Spring_Pin_1_8_in_OD_1_4_in_L_7_RIGID : Subsystem
  Spring_Pin_1_8_in_OD_1_4_in_L_8_RIGID : Subsystem
  Spring_Pin_1_8_in_OD_1_4_in_L_9_RIGID : Subsystem
  Standoff_1_RIGID : Subsystem
  Transform : sm_lib/Frames and Transforms/Rigid Transform  TranslationMethod=Cartesian  TranslationStandardOffset=0  TranslationLengthUnit=in  TranslationStandardAxis=+Z  TranslationCartesianOffset=frontParams.RigidTransform(422).translation  TranslationROffset=0  TranslationROffsetUnits=m  TranslationZOffset=0  TranslationZOffsetUnits=m  TranslationThetaOffset=0  TranslationThetaOffsetUnits=deg  RotationMethod=ArbitraryAxis  RotationAngleUnits=rad  RotationStandardAxis=+Z  RotationAngle=frontParams.RigidTransform(422).angle  RotationArbitraryAxis=frontParams.RigidTransform(422).axis  FollAlignAxisA=+X  BaseAlignAxisA=+Y  FollAlignAxisB=+Y  BaseAlignAxisB=+Z  RotationSequenceAxes=FollowerAxes  RotationSequence=XYX  RotationSequenceAngles=[0 0 0]  RotationSequenceAnglesUnits=deg  RotationMatrix=[1 0 0; 0 1 0; 0 0 1]
  Washer_10_1_RIGID : Subsystem
  Washer_10_2_RIGID : Subsystem
  Washer_10_3_RIGID : Subsystem
  Washer_10_4_RIGID : Subsystem
  Washer_8_1_RIGID : Subsystem
  Washer_8_2_RIGID : Subsystem
  bulkheads5_1_RIGID : Subsystem
  bulkheads5_2_RIGID : Subsystem
  bulkheads5_3_RIGID : Subsystem
  bulkheads5_4_RIGID : Subsystem
  bulkheads5_5_RIGID : Subsystem
  bulkheads6_1_RIGID : Subsystem
  bulkheads6_2_RIGID : Subsystem
  bulkheads6_3_RIGID : Subsystem
  bulkheads6_4_RIGID : Subsystem
  bulkheads6_5_RIGID : Subsystem
  forward_torso_l_1_RIGID : Subsystem
  forward_torso_r_1_RIGID : Subsystem
  F : PMIOPort  Side=Left
  F2 : PMIOPort  Port=2  Side=Left
  F1 : PMIOPort  Port=3  Side=Right
  S2 : PMIOPort  Port=4  Side=Right
  S3 : PMIOPort  Port=5  Side=Right
  connections:
  Bracket_1_RIGID/LConn1 -- Hinge_1_RIGID/LConn1 -- Spacer_2_RIGID/LConn1 -- bulkheads5_3_RIGID/LConn1 -- bulkheads5_4_RIGID/LConn1 -- bulkheads5_5_RIGID/LConn1 -- bulkheads6_1_RIGID/LConn1 -- bulkheads6_2_RIGID/LConn1 -- bulkheads6_3_RIGID/LConn1 -- bulkheads6_4_RIGID/LConn1 -- bulkheads6_5_RIGID/LConn1 -- forward_torso_l_1_RIGID/LConn1 -- bulkheads5_2_RIGID/LConn1 -- forward_torso_r_1_RIGID/LConn3 -- bulkheads5_1_RIGID/LConn1 -- Washer_8_2_RIGID/LConn1 -- Washer_8_1_RIGID/LConn1 -- Washer_10_4_RIGID/LConn1 -- Washer_10_3_RIGID/LConn1 -- Washer_10_2_RIGID/LConn1 -- Washer_10_1_RIGID/LConn1 -- Standoff_1_RIGID/LConn1 -- Spring_Pin_1_8_in_OD_1_4_in_L_9_RIGID/LConn1 -- Spring_Pin_1_8_in_OD_1_4_in_L_8_RIGID/LConn1 -- Spring_Pin_1_8_in_OD_1_4_in_L_7_RIGID/LConn1 -- Spring_Pin_1_8_in_OD_1_4_in_L_6_RIGID/LConn1 -- Spring_Pin_1_8_in_OD_1_4_in_L_5_RIGID/LConn1 -- Spring_Pin_1_8_in_OD_1_4_in_L_4_RIGID/LConn1 -- Spring_Pin_1_8_in_OD_1_4_in_L_3_RIGID/LConn1 -- Spring_Pin_1_8_in_OD_1_4_in_L_2_RIGID/LConn1 -- Spring_Pin_1_8_in_OD_1_4_in_L_22_RIGID/LConn1 -- Spring_Pin_1_8_in_OD_1_4_in_L_21_RIGID/LConn1 -- Spring_Pin_1_8_in_OD_1_4_in_L_20_RIGID/LConn1 -- Spring_Pin_1_8_in_OD_1_4_in_L_1_RIGID/LConn1 -- Spring_Pin_1_8_in_OD_1_4_in_L_19_RIGID/LConn1 -- Spring_Pin_1_8_in_OD_1_4_in_L_18_RIGID/LConn1 -- Spring_Pin_1_8_in_OD_1_4_in_L_17_RIGID/LConn1 -- Spring_Pin_1_8_in_OD_1_4_in_L_16_RIGID/LConn1 -- Spring_Pin_1_8_in_OD_1_4_in_L_15_RIGID/LConn1 -- Spring_Pin_1_8_in_OD_1_4_in_L_14_RIGID/LConn1 -- Spring_Pin_1_8_in_OD_1_4_in_L_13_RIGID/LConn1 -- Spring_Pin_1_8_in_OD_1_4_in_L_12_RIGID/LConn1 -- Spring_Pin_1_8_in_OD_1_4_in_L_11_RIGID/LConn1 -- Spring_Pin_1_8_in_OD_1_4_in_L_10_RIGID/LConn1 -- Spacer_1_RIGID/LConn1 -- Set_Screw_4_1_4_in_6_RIGID/LConn1 -- Set_Screw_4_1_4_in_5_RIGID/LConn1 -- Set_Screw_4_1_4_in_4_RIGID/LConn1 -- Set_Screw_4_1_4_in_3_RIGID/LConn1 -- Set_Screw_4_1_4_in_2_RIGID/LConn1 -- Set_Screw_4_1_4_in_1_RIGID/LConn1 -- Screw_8_1_2_in_2_RIGID/LConn1 -- Screw_8_1_2_in_1_RIGID/LConn1 -- Screw_10_3_4_in_4_RIGID/LConn1 -- Screw_10_3_4_in_3_RIGID/LConn1 -- Screw_10_3_4_in_2_RIGID/LConn1 -- Screw_10_3_4_in_1_RIGID/LConn1 -- Part_925_1_RIGID/LConn1 -- Part_924_1_RIGID/LConn1 -- Part_923_1_RIGID/LConn1 -- Part_855_1_RIGID/LConn1 -- Part_854_1_RIGID/LConn1 -- Part_853_1_RIGID/LConn1 -- Hinge_3_RIGID/LConn1 -- Hinge_2_RIGID/LConn1 -- Bracket_6_RIGID/LConn1 -- Bracket_5_RIGID/LConn1 -- Bracket_4_RIGID/LConn1 -- Bracket_3_RIGID/LConn1 -- Bracket_2_RIGID/LConn1
  forward_torso_r_1_RIGID/LConn2 -- F/RConn1
  Spacer_2_RIGID/LConn2 -- F1/RConn1
  Hinge_1_RIGID/LConn2 -- F2/RConn1
  Transform/RConn1 -- forward_torso_r_1_RIGID/LConn1
  ReferenceFrame/RConn1 -- Transform/LConn1
  S2/RConn1 -- forward_torso_r_1_RIGID/RConn1
  S3/RConn1 -- forward_torso_r_1_RIGID/RConn2
